simulink model "center_control"  (R2016a)
settings: Solver=VariableStepAuto  StartTime=0.0  StopTime=10.0  RelTol=1e-3
undefined symbols (not defined in the file): Angular, Linear
libraries: robotlib x3
settings Model: Creator=ece446  LastModifiedBy=ece446

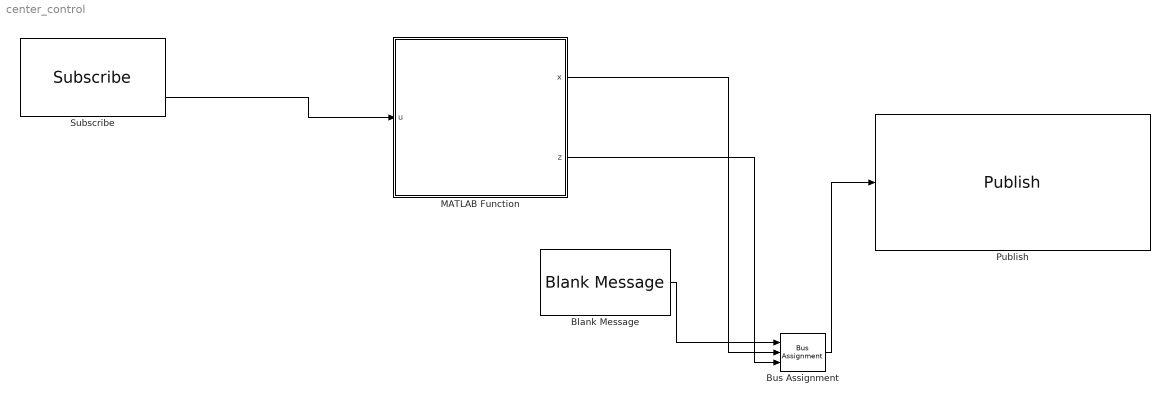
== system center_control ==
  Blank Message : robotlib/Blank Message  SourceLibraryInfo=This block requires Robotics System Toolbox  messageType=geometry_msgs/Twist  SampleTime=inf
  Bus Assignment : BusAssignment  AssignedSignals=Linear.X,Angular.Z
  MATLAB Function : MATLAB Function  TreatAsAtomicUnit=on
  Publish : robotlib/Publish  SourceLibraryInfo=This block requires Robotics System Toolbox  topicSource=Select from ROS network  topic=/catvehicle/cmd_vel  messageType=geometry_msgs/Twist  messageQueueLength=1
  Subscribe : robotlib/Subscribe  SourceLibraryInfo=This block requires Robotics System Toolbox  topicSource=Select from ROS network  topic=/detections  messageType=geometry_msgs/PolygonStamped  sampleTime=-1  messageQueueLength=1
  wires:
  Subscribe/2 -> MATLAB Function/1(u)
  Blank Message/1 -> Bus Assignment/1
  Bus Assignment/1 -> Publish/1
  MATLAB Function/1(x) -> Bus Assignment/2
  MATLAB Function/2(z) -> Bus Assignment/3

== matlab function center_control/MATLAB Function ==
  data: u input; x output; z output
function [x,z]= fcn(u)
%#codegen
x = 0;
z = 0;
